simulink model "Lab1_session5_PID"  (R2022b)
settings: Solver=VariableStepAuto  StartTime=0.0  StopTime=10  RelTol=1e-3
settings Model: Creator=Dell  LastModifiedBy=Dell

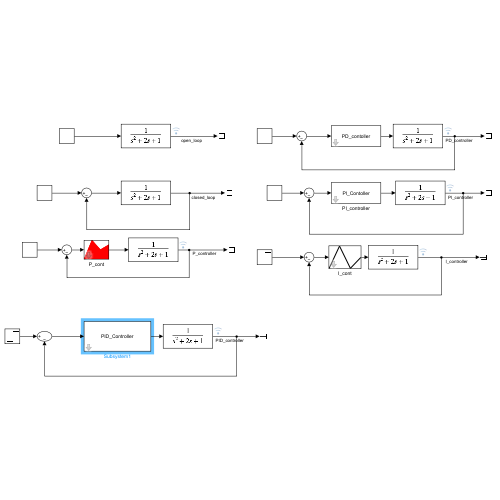
[thumbnail: Simulink's stored preview of the top-level diagram]
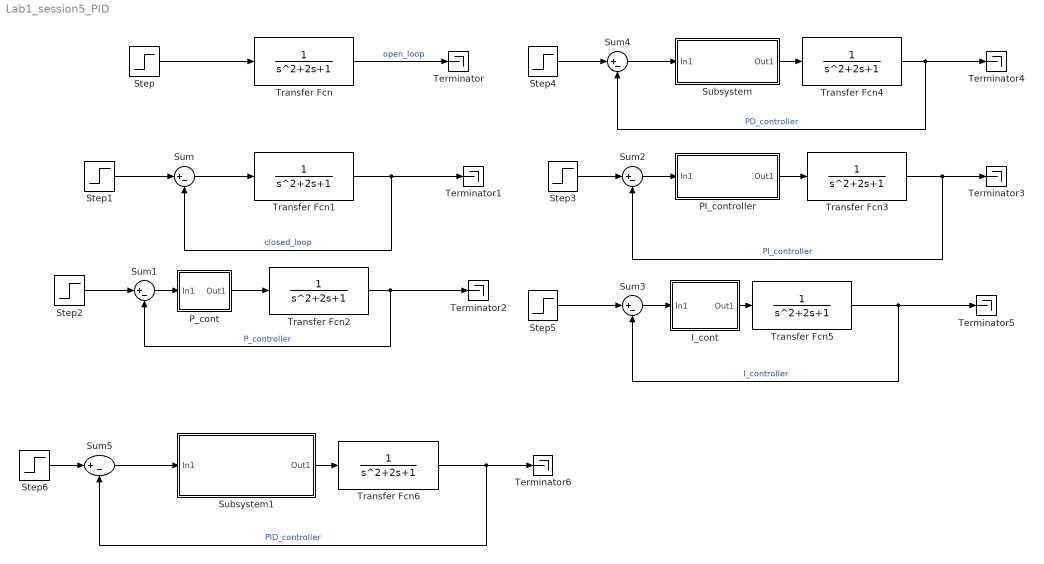
== system Lab1_session5_PID ==
  I_cont : Subsystem  mask{KI=2}
      mask Display:
      | plot([10 20 30 40], [10 20 10 15]);
      | color('red');
  PI_controller : Subsystem  mask{KP=1, KI=1}
      mask Display:
      | disp('PI_Contoller');
      | color('red');
  P_cont : Subsystem  mask{KP=2}
      mask Display:
      | patch([0 10 20 30 30 0], [10 30 20 25 10 10], [1 0 0]);
      | patch([0 10 20 30 30 0], [10 30 20 25 10 10], [1 0 0]);
  Step{,1..6} (7 alike) : Step  SampleTime=0
  Subsystem : Subsystem  mask{KP=1, KD=1}
      mask Display: disp('PD_contoller');
  Subsystem1 : Subsystem  mask{KP=19, KI=1.9, KD=10}
      mask Display: disp('PID_Controller');
  Sum{,1..5} (6 alike) : Sum  Inputs=|+-
  Terminator{,1..6} (7 alike) : Terminator
  Transfer Fcn{,1..6} (7 alike) : TransferFcn
  wires:
  Transfer Fcn/1 -> Terminator/1  "open_loop"
  Step/1 -> Transfer Fcn/1
  Transfer Fcn1/1 -> Terminator1/1, Sum/2  "closed_loop"
  Step1/1 -> Sum/1
  Sum/1 -> Transfer Fcn1/1
  Transfer Fcn2/1 -> Sum1/2, Terminator2/1  "P_controller"
  Step2/1 -> Sum1/1
  P_cont/1(Out1) -> Transfer Fcn2/1
  Sum1/1 -> P_cont/1(In1)
  Sum3/1 -> I_cont/1(In1)
  I_cont/1(Out1) -> Transfer Fcn5/1
  Step5/1 -> Sum3/1
  Transfer Fcn5/1 -> Terminator5/1, Sum3/2  "I_controller"
  Transfer Fcn3/1 -> Sum2/2, Terminator3/1  "PI_controller"
  Step3/1 -> Sum2/1
  Sum2/1 -> PI_controller/1(In1)
  PI_controller/1(Out1) -> Transfer Fcn3/1
  Step4/1 -> Sum4/1
  Sum4/1 -> Subsystem/1(In1)
  Subsystem/1(Out1) -> Transfer Fcn4/1
  Transfer Fcn4/1 -> Terminator4/1, Sum4/2  "PD_controller"
  Sum5/1 -> Subsystem1/1(In1)
  Step6/1 -> Sum5/1
  Subsystem1/1(Out1) -> Transfer Fcn6/1
  Transfer Fcn6/1 -> Terminator6/1, Sum5/2  "PID_controller"

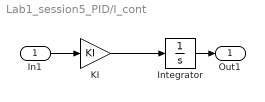
== system Lab1_session5_PID/I_cont ==
  In1 : Inport
  Integrator : Integrator
  KI : Gain  Gain=KI
  Out1 : Outport
  wires:
  KI/1 -> Integrator/1
  In1/1 -> KI/1
  Integrator/1 -> Out1/1

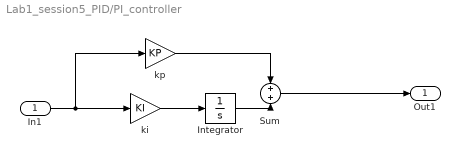
== system Lab1_session5_PID/PI_controller ==
  In1 : Inport
  Integrator : Integrator
  Sum : Sum
  ki : Gain  Gain=KI
  kp : Gain  Gain=KP
  Out1 : Outport
  wires:
  ki/1 -> Integrator/1
  kp/1 -> Sum/1
  Integrator/1 -> Sum/2
  Sum/1 -> Out1/1
  In1/1 -> kp/1, ki/1

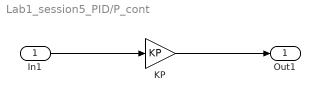
== system Lab1_session5_PID/P_cont ==
  In1 : Inport
  KP : Gain  Gain=KP
  Out1 : Outport
  wires:
  In1/1 -> KP/1
  KP/1 -> Out1/1

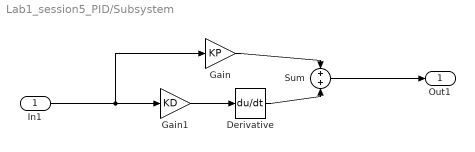
== system Lab1_session5_PID/Subsystem ==
  In1 : Inport
  Derivative : Derivative
  Gain : Gain  Gain=KP
  Gain1 : Gain  Gain=KD
  Sum : Sum
  Out1 : Outport
  wires:
  Gain1/1 -> Derivative/1
  Gain/1 -> Sum/1
  Derivative/1 -> Sum/2
  Sum/1 -> Out1/1
  In1/1 -> Gain/1, Gain1/1

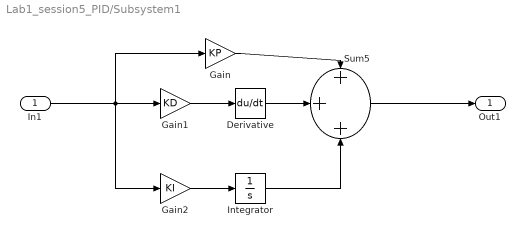
== system Lab1_session5_PID/Subsystem1 ==
  In1 : Inport
  Derivative : Derivative
  Gain : Gain  Gain=KP
  Gain1 : Gain  Gain=KD
  Gain2 : Gain  Gain=KI
  Integrator : Integrator
  Sum5 : Sum  Inputs=+++
  Out1 : Outport
  wires:
  Gain1/1 -> Derivative/1
  Integrator/1 -> Sum5/3
  Gain2/1 -> Integrator/1
  Gain/1 -> Sum5/1
  Derivative/1 -> Sum5/2
  In1/1 -> Gain/1, Gain2/1, Gain1/1
  Sum5/1 -> Out1/1
